simulink model "manipulator_ovladani"  (R2023a)
settings: Solver=ode45  StartTime=0  StopTime=10  FixedStep=.01  RelTol=1e-3  EnableMultiTasking=on
values from neighbouring files (symbols this model uses):
  qic = Deval*q    [parsys.m]
settings Model: Creator=Janfron  LastModifiedBy=MarekUser
settings SolverCC: AlgebraicLoopSolver=TrustRegion
settings DataIOCC: SaveFormat=Array  SignalLoggingSaveFormat=ModelDataLogs  ReturnWorkspaceOutputs=off  SignalLoggingName=sigsOut
settings OptimizationCC: BooleanDataType=off  ExpressionDepthLimit=2147483647  InitFltsAndDblsToZero=on  LifeSpan=inf
settings DebuggingCC: SaveWithParameterizedLinksMsg=none  UnderspecifiedInitializationDetection=Classic  MergeDetectMultiDrivingBlocksExec=none  SignalResolutionControl=TryResolveAllWithWarning  MultiTaskDSMMsg=warning  MultiTaskCondExecSysMsg=none  FcnCallInpInsideContextMsg=warning  UnconnectedInputMsg=warning  UnconnectedOutputMsg=warning  UnconnectedLineMsg=warning  StateNameClashWarn=warning  SFUnexpectedBacktrackingDiag=warning  SFNoUnconditionalDefaultTransitionDiag=warning  SFExecutionAtInitializationDiag=none  ArithmeticOperatorsInVariantConditions=warning
settings HardwareCC: ProdBitPerPointer=32  ProdBitPerSizeT=32  ProdBitPerPtrDiffT=32  ProdLargestAtomicFloat=None  ProdIntDivRoundTo=Undefined  ProdEndianess=Unspecified  ProdWordSize=32  ProdHWDeviceType=32-bit Generic  TargetUnknown=on
settings ModelReferenceCC: EnableRefExpFcnMdlSchedulingChecks=on  PropagateSignalLabelsOutOfModel=off
settings SFSimCC: SimUseLocalCustomCode=off  CustomCodeUndefinedFunction=UseInterfaceOnly
settings RTWCC: RTWUseLocalCustomCode=off
settings CodeAppCC: StateflowObjectComments=on
settings GRTTargetCC: TargetFcnLib=ansi_tfl_tmw.mat  TargetLangStandard=C89/C90 (ANSI)  CombineOutputUpdateFcns=off  GRTInterface=on
settings ConfigComp: CovMetricSettings=dw  CovSaveCumulativeToWorkspaceVar=on  CovSaveSingleToWorkspaceVar=on  CovExternalEMLEnable=off

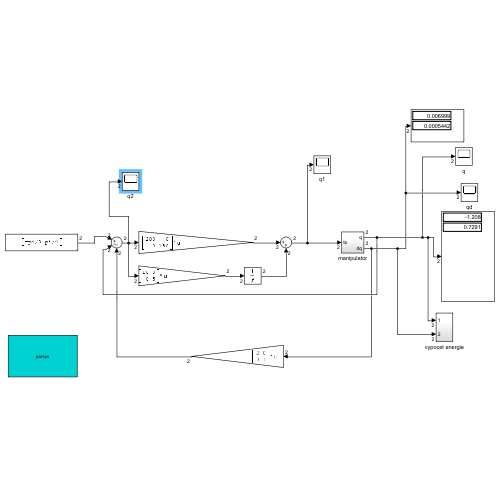
[thumbnail: Simulink's stored preview of the top-level diagram]
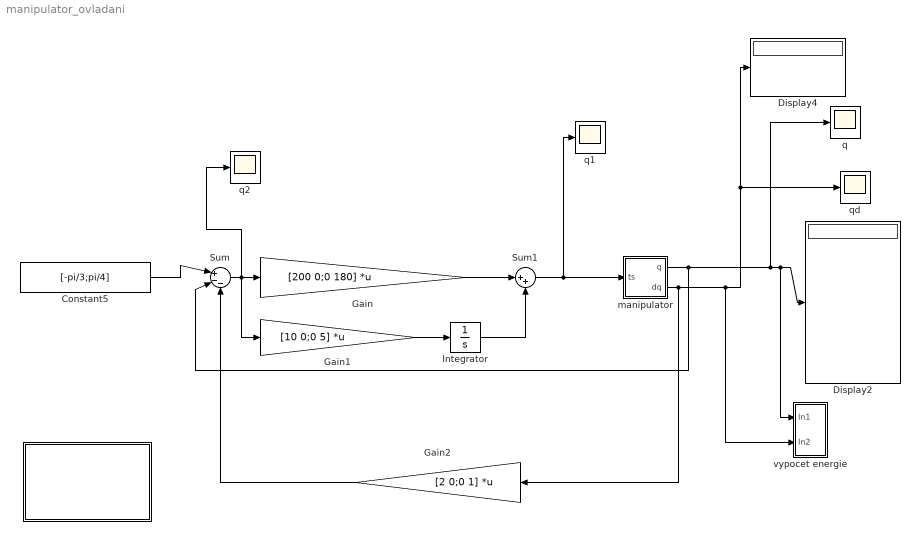
== system manipulator_ovladani ==
  " " : Subsystem  mask{Parameter1=[]}
      mask prompts: Parameter1 "eval('parsys')"
      settings: OpenFcn=parsys
      mask Display: disp('parsys')
  Constant5 : Constant  Value=[-pi/3;pi/4]
  Display2 : Display
  Display4 : Display
  Gain : Gain  Gain=[200 0;0 180]  Multiplication=Matrix(K*u)
  Gain1 : Gain  Gain=[10 0;0 5]  Multiplication=Matrix(K*u)
  Gain2 : Gain  Gain=[2 0;0 1]  Multiplication=Matrix(K*u)
  Integrator : Integrator
  Sum : Sum  Inputs=|+--
  Sum1 : Sum  Inputs=|++
  manipulator : Subsystem
  q : Scope
  q1 : Scope
  q2 : Scope
  qd : Scope
  vypocet energie : Subsystem
  wires:
  manipulator/1(q) -> Sum/2, Display2/1, vypocet energie/1(In1), q/1
  manipulator/2(dq) -> Gain2/1, Display4/1, qd/1, vypocet energie/2(In2)
  Sum/1 -> q2/1, Gain1/1, Gain/1
  Constant5/1 -> Sum/1
  Gain/1 -> Sum1/1
  Sum1/1 -> q1/1, manipulator/1(ts)
  Integrator/1 -> Sum1/2
  Gain1/1 -> Integrator/1
  Gain2/1 -> Sum/3

== system manipulator_ovladani/  ==

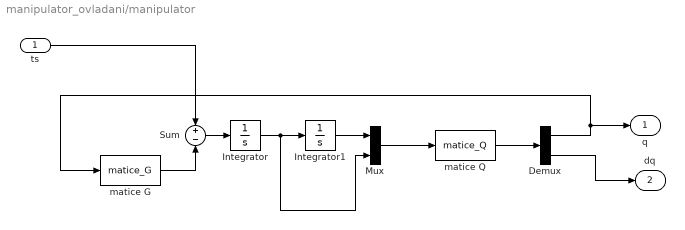
== system manipulator_ovladani/manipulator ==
  ts : Inport
  Demux : Demux  Outputs=[2 2]
      settings: DisplayOption=none
  Integrator : Integrator
  Integrator1 : Integrator  InitialCondition=qic
  Mux : Mux  Inputs=[2 2]
  Sum : Sum  Inputs=+-  InputSameDT=on  SaturateOnIntegerOverflow=on  OutDataTypeStr=Inherit: Same as first input
  matice G : MATLABFcn  MATLABFcn=matice_G
  matice Q : MATLABFcn  MATLABFcn=matice_Q
  q : Outport  VectorParamsAs1DForOutWhenUnconnected=off
  dq : Outport  Port=2  VectorParamsAs1DForOutWhenUnconnected=off
  wires:
  Integrator/1 -> Integrator1/1, Mux/2
  Mux/1 -> matice Q/1
  Sum/1 -> Integrator/1
  ts/1 -> Sum/1
  Demux/1 -> q/1, matice G/1
  Demux/2 -> dq/1
  matice G/1 -> Sum/2
  Integrator1/1 -> Mux/1
  matice Q/1 -> Demux/1

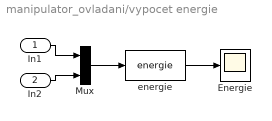
== system manipulator_ovladani/vypocet energie ==
  In1 : Inport
  In2 : Inport  Port=2
  Energie : Scope
  Mux : Mux  Inputs=[2 2]
  energie : MATLABFcn  MATLABFcn=energie  OutputDimensions=3
  wires:
  In2/1 -> Mux/2
  In1/1 -> Mux/1
  Mux/1 -> energie/1
  energie/1 -> Energie/1
